simulink model "ex3_s"  (R2020a)
settings: Solver=VariableStepAuto  StartTime=0.0  StopTime=20  RelTol=1e-3
undefined symbols (not defined in the file or in its folder): dz, nz

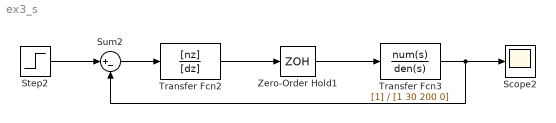
== system ex3_s ==
  Scope2 : Scope
  Step2 : Step  SampleTime=0.1
  Sum2 : Sum  Inputs=|+-  SampleTime=0.1
  Transfer Fcn2 : TransferFcn  Numerator=[nz]  Denominator=[dz]
  Transfer Fcn3 : TransferFcn  Denominator=[1 30 200 0]
  Zero-Order Hold1 : ZeroOrderHold  SampleTime=-1
  wires:
  Step2/1 -> Sum2/1
  Transfer Fcn3/1 -> Sum2/2, Scope2/1
  Sum2/1 -> Transfer Fcn2/1
  Transfer Fcn2/1 -> Zero-Order Hold1/1
  Zero-Order Hold1/1 -> Transfer Fcn3/1
